simulink model "cartpole_pd_simulink"  (R2025a)
settings: Solver=ode45  StartTime=0.0  StopTime=5  MaxStep=0.001  RelTol=1e-3
values from neighbouring files (symbols this model uses):
  Fmax = 50    [auto_tune_pid.m]    (also in setup_lqr.m; setup_pd.m; setup_pid.m)
  Kd = 15    [setup_pd.m]    (also in setup_pid.m = 5)
  Kp = 80    [setup_pd.m]    (also in setup_pid.m = 120)
settings Model: Creator=Lee  LastModifiedBy=Lee

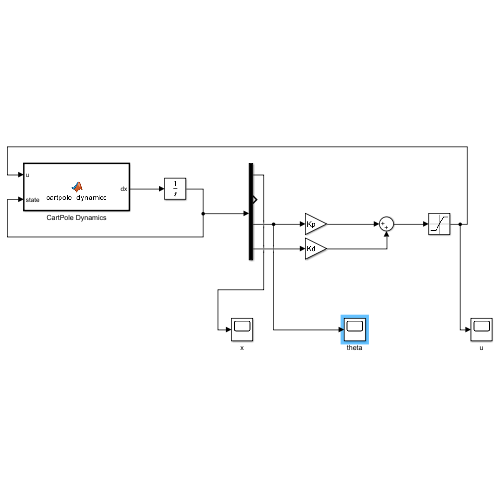
[thumbnail: Simulink's stored preview of the top-level diagram]
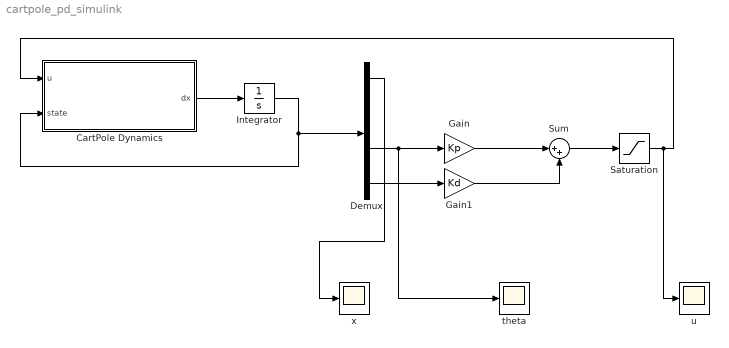
== system cartpole_pd_simulink ==
  CartPole Dynamics : MATLAB Function  TreatAsAtomicUnit=on
  Demux : Demux
  Gain : Gain  Gain=Kp
  Gain1 : Gain  Gain=Kd
  Integrator : Integrator  InitialCondition=[0; 0; deg2rad(5); 0]
  Saturation : Saturate  UpperLimit=Fmax  LowerLimit=-Fmax
  Sum : Sum  Inputs=|++
  theta : Scope
      settings: ActiveDisplayYMinimum=-0.010908307824964558  ActiveDisplayYMaximum=0.098174770424681035
  u : Scope
      settings: ActiveDisplayYMinimum=-1.0322291290093859  ActiveDisplayYMaximum=7.8717110231980625  DataLoggingVariableName=ScopeData2
  x : Scope
      settings: ActiveDisplayYMinimum=-0.11751994105742443  ActiveDisplayYMaximum=1.0576794695168201
  wires:
  CartPole Dynamics/1(dx) -> Integrator/1
  Integrator/1 -> Demux/1, CartPole Dynamics/2(state)
  Demux/3 -> theta/1, Gain/1
  Demux/4 -> Gain1/1
  Gain/1 -> Sum/1
  Gain1/1 -> Sum/2
  Sum/1 -> Saturation/1
  Saturation/1 -> u/1, CartPole Dynamics/1(u)
  Demux/1 -> x/1

== matlab function cartpole_pd_simulink/CartPole Dynamics ==
  data: u input; dx output; state input
function dx = cartpole_dynamics(u, state)

M = 1.0;
m = 0.1;
l = 0.5;
g = 9.8;

x = state(1);
x_dot = state(2);
theta = state(3);
theta_dot = state(4);

den = M + m*sin(theta)^2;

x_ddot = (u + m * sin(theta) * (l * theta_dot^2 - g * cos(theta))) / den;

theta_ddot = (-u * cos(theta) - m * l * theta_dot^2 * sin(theta) * cos(theta) + (M + m) * g * sin(theta)) / (l * den);

dx = zeros(4,1);
dx(1) = x_dot;
dx(2) = x_ddot;
dx(3) = theta_dot;
dx(4) = theta_ddot;

end
